simulink model "sm_mp1_re"  (R2023b)
settings: Solver=VariableStepAuto  StartTime=0.0  StopTime=10.0  RelTol=1e-3
undefined symbols (not defined in the file): A_eval, B_eval, k
settings Model: Creator=yonathan  LastModifiedBy=yonathan
settings DataIOCC: Refine=10

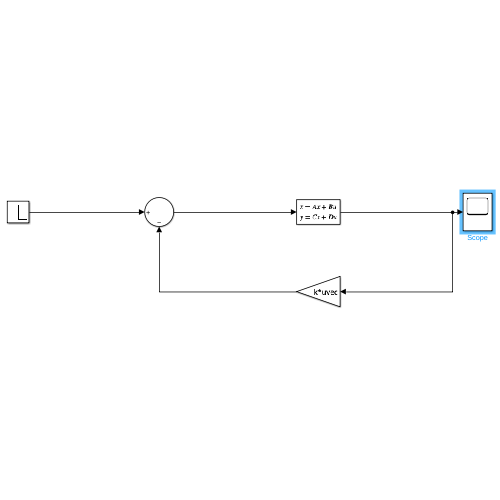
[thumbnail: Simulink's stored preview of the top-level diagram]
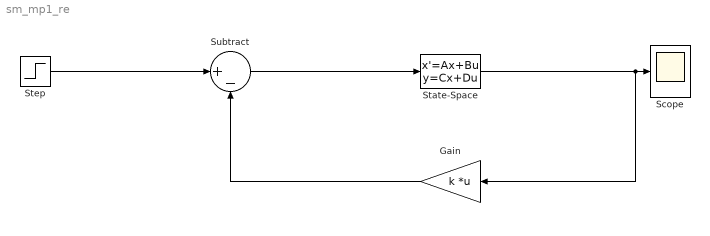
== system sm_mp1_re ==
  Gain : Gain  Gain=k  Multiplication=Matrix(K*u) (u vector)
  Scope : Scope
  State-Space : StateSpace  A=A_eval  B=B_eval  C=eye(6)  D=zeros(6,1)  InitialCondition=[0 0 0 0 0.05 0]
  Step : Step  Before=0.05  After=0  SampleTime=0
  Subtract : Sum  Inputs=|+-
  wires:
  Gain/1 -> Subtract/2
  Subtract/1 -> State-Space/1
  State-Space/1 -> Gain/1, Scope/1
  Step/1 -> Subtract/1
